simulink model "Model"  (R2017a)
settings: Solver=VariableStepAuto  StartTime=0.0  StopTime=10.0  RelTol=1e-3
settings Model: Creator=gabriele  LastModifiedBy=gabriele

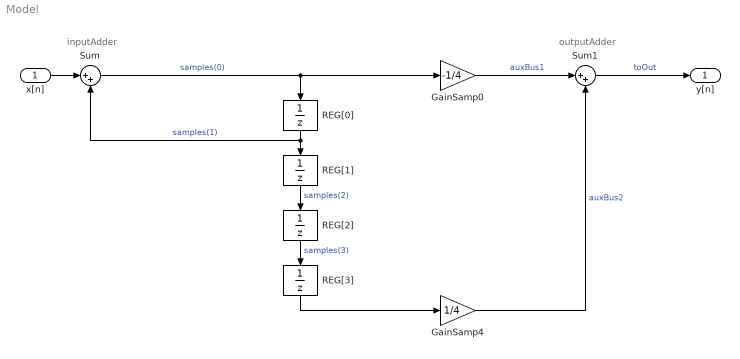
== system Model ==
  note: outputAdder
  note: inputAdder
  x[n] : Inport
  GainSamp0 : Gain  Gain=-1/4
  GainSamp4 : Gain  Gain=1/4
  REG[0] : UnitDelay  SampleTime=-1
  REG[1] : UnitDelay  SampleTime=-1
  REG[2] : UnitDelay  SampleTime=-1
  REG[3] : UnitDelay  SampleTime=-1
  Sum : Sum  Inputs=|++
  Sum1 : Sum  Inputs=|++
  y[n] : Outport
  wires:
  Sum/1 -> REG[0]/1, GainSamp0/1  "samples(0)"
  REG[0]/1 -> Sum/2, REG[1]/1  "samples(1)"
  REG[1]/1 -> REG[2]/1  "samples(2)"
  REG[2]/1 -> REG[3]/1  "samples(3)"
  GainSamp0/1 -> Sum1/1  "auxBus1"
  REG[3]/1 -> GainSamp4/1
  GainSamp4/1 -> Sum1/2  "auxBus2"
  x[n]/1 -> Sum/1
  Sum1/1 -> y[n]/1  "toOut"
